simulink library "utilities"  (R2016b)
settings: Solver=VariableStepAuto  StartTime=0.0  StopTime=10.0  RelTol=1e-3
settings Model: Creator=bclzl  LastModifiedBy=bclzl

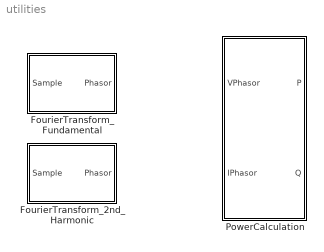
== system utilities ==
  FourierTransform_2nd_Harmonic : Subsystem
  FourierTransform_Fundamental : Subsystem
  PowerCalculation : Subsystem

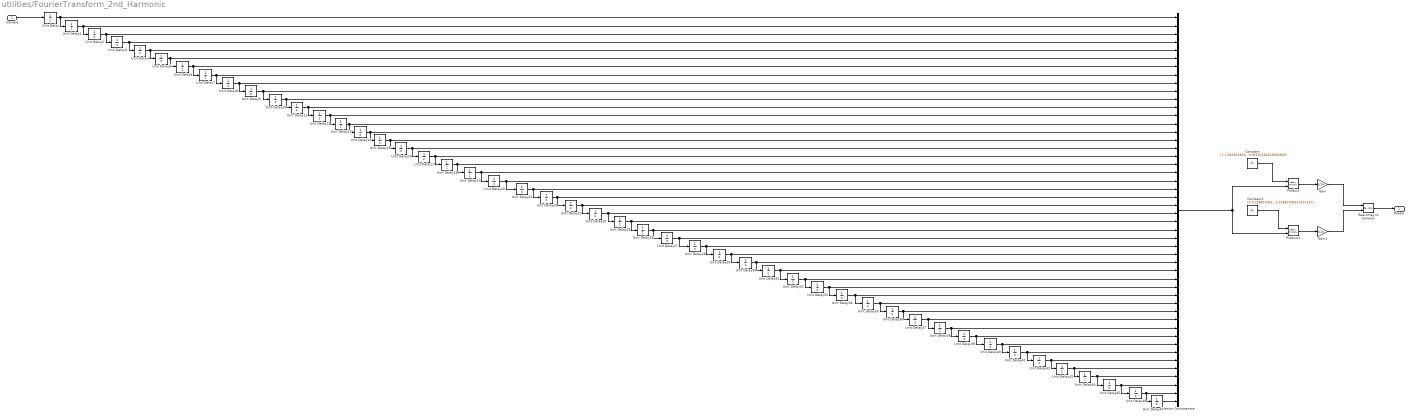
== system utilities/FourierTransform_2nd_Harmonic ==
  Sample : Inport
  Constant : Constant  Value=[1 0.96592582628906831 0.86602540378443871 0.70710678118654757 0.50000000000000011 0.25881904510252074 6.123233995736766E-17 -0.25881904510252063 -0.49999999999999978 -0.70710678118654746 -0.86602540378443871 -0.9659258262890682 -1 -0.96592582628906831 -0.86602540378443882 -0.70710678118654791 -0.50000000000000044 -0.25881904510252063 -1.8369701987210297E-16 0.2588190451025203 0.50000000000000011 0.70710678118654735 0.86602540378443837 0.96592582628906809 1 0.96592582628906831 0.86602540378443871 0.70710678118654757 0.50000000000000011 0.25881904510252074 6.123233995736766E-17 -0.25881904510252063 -0.49999999999999978 -0.70710678118654746 -0.86602540378443871 -0.9659258262890682 -1 -0.96592582628906831 -0.86602540378443882 -0.70710678118654791 -0.50000000000000044 -0.25881904510252063 -1.8369701987210297E-16 0.2588190451025203 0.50000000000000011 0.70710678118654735 0.86602540378443837 0.96592582628906809]  VectorParams1D=off
  Constant1 : Constant  Value=[0 0.25881904510252074 0.49999999999999994 0.70710678118654746 0.8660254037844386 0.96592582628906831 1 0.96592582628906831 0.86602540378443871 0.70710678118654757 0.49999999999999994 0.258819045102521 1.2246467991473532E-16 -0.25881904510252079 -0.49999999999999972 -0.70710678118654713 -0.86602540378443849 -0.96592582628906831 -1 -0.96592582628906842 -0.8660254037844386 -0.70710678118654768 -0.50000000000000044 -0.25881904510252157 0 0.25881904510252074 0.49999999999999994 0.70710678118654746 0.8660254037844386 0.96592582628906831 1 0.96592582628906831 0.86602540378443871 0.70710678118654757 0.49999999999999994 0.258819045102521 1.2246467991473532E-16 -0.25881904510252079 -0.49999999999999972 -0.70710678118654713 -0.86602540378443849 -0.96592582628906831 -1 -0.96592582628906842 -0.8660254037844386 -0.70710678118654768 -0.50000000000000044 -0.25881904510252157]  VectorParams1D=off
  Gain : Gain  Gain=1/24
  Gain1 : Gain  Gain=1/24
  Product : Product  Multiplication=Matrix(*)
  Product1 : Product  Multiplication=Matrix(*)
  Real-Imag to Complex : RealImagToComplex
  Unit Delay{,1..47} (48 alike) : UnitDelay  SampleTime=-1
  Vector Concatenate : Concatenate  NumInputs=48  Mode=Multidimensional array
  Phasor : Outport
  wires:
  Real-Imag to Complex/1 -> Phasor/1
  Gain1/1 -> Real-Imag to Complex/2
  Product1/1 -> Gain1/1
  Constant1/1 -> Product1/1
  Gain/1 -> Real-Imag to Complex/1
  Product/1 -> Gain/1
  Constant/1 -> Product/1
  Unit Delay29/1 -> Unit Delay30/1, Vector Concatenate/30
  Unit Delay30/1 -> Unit Delay31/1, Vector Concatenate/31
  Unit Delay26/1 -> Unit Delay27/1, Vector Concatenate/27
  Unit Delay27/1 -> Unit Delay28/1, Vector Concatenate/28
  Unit Delay28/1 -> Unit Delay29/1, Vector Concatenate/29
  Unit Delay41/1 -> Unit Delay42/1, Vector Concatenate/42
  Unit Delay42/1 -> Unit Delay43/1, Vector Concatenate/43
  Unit Delay43/1 -> Unit Delay44/1, Vector Concatenate/44
  Unit Delay46/1 -> Unit Delay47/1, Vector Concatenate/47
  Unit Delay40/1 -> Unit Delay41/1, Vector Concatenate/41
  Unit Delay47/1 -> Vector Concatenate/48
  Sample/1 -> Unit Delay/1
  Unit Delay1/1 -> Unit Delay2/1, Vector Concatenate/2
  Vector Concatenate/1 -> Product/2, Product1/2
  Unit Delay5/1 -> Unit Delay6/1, Vector Concatenate/6
  Unit Delay19/1 -> Unit Delay20/1, Vector Concatenate/20
  Unit Delay20/1 -> Unit Delay21/1, Vector Concatenate/21
  Unit Delay21/1 -> Unit Delay22/1, Vector Concatenate/22
  Unit Delay24/1 -> Unit Delay25/1, Vector Concatenate/25
  Unit Delay23/1 -> Unit Delay24/1, Vector Concatenate/24
  Unit Delay22/1 -> Unit Delay23/1, Vector Concatenate/23
  Unit Delay9/1 -> Unit Delay10/1, Vector Concatenate/10
  Unit Delay25/1 -> Unit Delay26/1, Vector Concatenate/26
  Unit Delay13/1 -> Unit Delay14/1, Vector Concatenate/14
  Unit Delay6/1 -> Unit Delay7/1, Vector Concatenate/7
  Unit Delay4/1 -> Unit Delay5/1, Vector Concatenate/5
  Unit Delay14/1 -> Unit Delay15/1, Vector Concatenate/15
  Unit Delay17/1 -> Unit Delay18/1, Vector Concatenate/18
  Unit Delay16/1 -> Unit Delay17/1, Vector Concatenate/17
  Unit Delay18/1 -> Unit Delay19/1, Vector Concatenate/19
  Unit Delay15/1 -> Unit Delay16/1, Vector Concatenate/16
  Unit Delay8/1 -> Unit Delay9/1, Vector Concatenate/9
  Unit Delay3/1 -> Unit Delay4/1, Vector Concatenate/4
  Unit Delay2/1 -> Unit Delay3/1, Vector Concatenate/3
  Unit Delay12/1 -> Unit Delay13/1, Vector Concatenate/13
  Unit Delay10/1 -> Unit Delay11/1, Vector Concatenate/11
  Unit Delay11/1 -> Unit Delay12/1, Vector Concatenate/12
  Unit Delay/1 -> Unit Delay1/1, Vector Concatenate/1
  Unit Delay37/1 -> Unit Delay38/1, Vector Concatenate/38
  Unit Delay38/1 -> Unit Delay39/1, Vector Concatenate/39
  Unit Delay39/1 -> Unit Delay40/1, Vector Concatenate/40
  Unit Delay34/1 -> Unit Delay35/1, Vector Concatenate/35
  Unit Delay35/1 -> Unit Delay36/1, Vector Concatenate/36
  Unit Delay36/1 -> Unit Delay37/1, Vector Concatenate/37
  Unit Delay33/1 -> Unit Delay34/1, Vector Concatenate/34
  Unit Delay32/1 -> Unit Delay33/1, Vector Concatenate/33
  Unit Delay44/1 -> Unit Delay45/1, Vector Concatenate/45
  Unit Delay45/1 -> Unit Delay46/1, Vector Concatenate/46
  Unit Delay7/1 -> Unit Delay8/1, Vector Concatenate/8
  Unit Delay31/1 -> Unit Delay32/1, Vector Concatenate/32

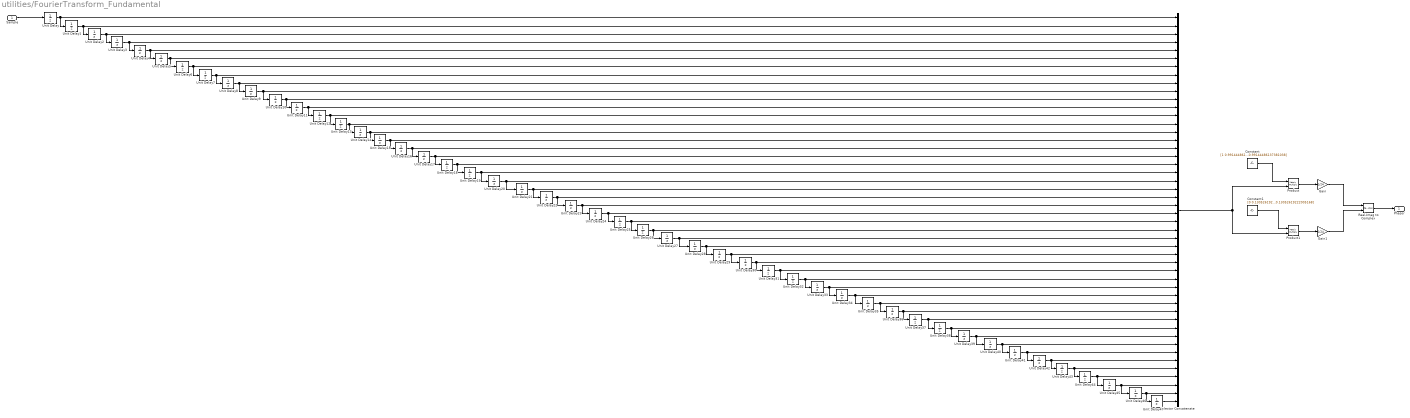
== system utilities/FourierTransform_Fundamental ==
  Sample : Inport
  Constant : Constant  Value=[1 0.99144486137381038 0.96592582628906831 0.92387953251128674 0.86602540378443871 0.79335334029123517 0.70710678118654757 0.60876142900872066 0.50000000000000011 0.38268343236508984 0.25881904510252074 0.13052619222005171 6.123233995736766E-17 -0.13052619222005138 -0.25881904510252085 -0.38268343236508973 -0.49999999999999978 -0.60876142900872066 -0.70710678118654746 -0.793353340291235 -0.86602540378443871 -0.92387953251128674 -0.9659258262890682 -0.99144486137381038 -1 -0.99144486137381038 -0.96592582628906842 -0.92387953251128685 -0.8660254037844386 -0.79335334029123539 -0.70710678118654768 -0.60876142900872088 -0.50000000000000044 -0.38268343236509034 -0.25881904510252063 -0.13052619222005163 -1.8369701987210297E-16 0.13052619222005127 0.2588190451025203 0.38268343236509 0.50000000000000011 0.60876142900872054 0.70710678118654735 0.79335334029123494 0.86602540378443837 0.92387953251128652 0.96592582628906831 0.99144486137381038]  VectorParams1D=off
  Constant1 : Constant  Value=[0 0.13052619222005157 0.25881904510252074 0.38268343236508978 0.49999999999999994 0.60876142900872066 0.70710678118654746 0.79335334029123517 0.8660254037844386 0.92387953251128674 0.96592582628906831 0.99144486137381038 1 0.99144486137381049 0.96592582628906831 0.92387953251128674 0.86602540378443871 0.79335334029123517 0.70710678118654757 0.60876142900872088 0.49999999999999994 0.38268343236508989 0.258819045102521 0.13052619222005157 1.2246467991473532E-16 -0.13052619222005177 -0.25881904510252035 -0.38268343236508967 -0.50000000000000011 -0.60876142900872032 -0.70710678118654746 -0.79335334029123494 -0.86602540378443849 -0.92387953251128652 -0.96592582628906831 -0.99144486137381038 -1 -0.99144486137381049 -0.96592582628906842 -0.92387953251128663 -0.8660254037844386 -0.79335334029123517 -0.70710678118654768 -0.60876142900872088 -0.50000000000000044 -0.38268343236509039 -0.25881904510252068 -0.13052619222005168]  VectorParams1D=off
  Gain : Gain  Gain=1/24
  Gain1 : Gain  Gain=1/24
  Product : Product  Multiplication=Matrix(*)
  Product1 : Product  Multiplication=Matrix(*)
  Real-Imag to Complex : RealImagToComplex
  Unit Delay{,1..47} (48 alike) : UnitDelay  SampleTime=-1
  Vector Concatenate : Concatenate  NumInputs=48  Mode=Multidimensional array
  Phasor : Outport
  wires:
  Unit Delay31/1 -> Vector Concatenate/32, Unit Delay32/1
  Unit Delay7/1 -> Vector Concatenate/8, Unit Delay8/1
  Unit Delay45/1 -> Vector Concatenate/46, Unit Delay46/1
  Unit Delay44/1 -> Vector Concatenate/45, Unit Delay45/1
  Unit Delay32/1 -> Vector Concatenate/33, Unit Delay33/1
  Unit Delay33/1 -> Vector Concatenate/34, Unit Delay34/1
  Unit Delay36/1 -> Vector Concatenate/37, Unit Delay37/1
  Unit Delay35/1 -> Vector Concatenate/36, Unit Delay36/1
  Unit Delay34/1 -> Vector Concatenate/35, Unit Delay35/1
  Unit Delay39/1 -> Vector Concatenate/40, Unit Delay40/1
  Unit Delay38/1 -> Vector Concatenate/39, Unit Delay39/1
  Unit Delay37/1 -> Vector Concatenate/38, Unit Delay38/1
  Unit Delay/1 -> Vector Concatenate/1, Unit Delay1/1
  Unit Delay11/1 -> Vector Concatenate/12, Unit Delay12/1
  Unit Delay10/1 -> Vector Concatenate/11, Unit Delay11/1
  Unit Delay12/1 -> Vector Concatenate/13, Unit Delay13/1
  Unit Delay2/1 -> Vector Concatenate/3, Unit Delay3/1
  Unit Delay3/1 -> Vector Concatenate/4, Unit Delay4/1
  Unit Delay8/1 -> Vector Concatenate/9, Unit Delay9/1
  Unit Delay15/1 -> Vector Concatenate/16, Unit Delay16/1
  Unit Delay18/1 -> Vector Concatenate/19, Unit Delay19/1
  Unit Delay16/1 -> Vector Concatenate/17, Unit Delay17/1
  Unit Delay17/1 -> Vector Concatenate/18, Unit Delay18/1
  Unit Delay14/1 -> Vector Concatenate/15, Unit Delay15/1
  Unit Delay4/1 -> Vector Concatenate/5, Unit Delay5/1
  Unit Delay6/1 -> Vector Concatenate/7, Unit Delay7/1
  Unit Delay13/1 -> Vector Concatenate/14, Unit Delay14/1
  Unit Delay25/1 -> Vector Concatenate/26, Unit Delay26/1
  Unit Delay9/1 -> Vector Concatenate/10, Unit Delay10/1
  Unit Delay22/1 -> Vector Concatenate/23, Unit Delay23/1
  Unit Delay23/1 -> Vector Concatenate/24, Unit Delay24/1
  Unit Delay24/1 -> Vector Concatenate/25, Unit Delay25/1
  Unit Delay21/1 -> Vector Concatenate/22, Unit Delay22/1
  Unit Delay20/1 -> Vector Concatenate/21, Unit Delay21/1
  Unit Delay19/1 -> Vector Concatenate/20, Unit Delay20/1
  Unit Delay5/1 -> Vector Concatenate/6, Unit Delay6/1
  Vector Concatenate/1 -> Product1/2, Product/2
  Unit Delay1/1 -> Vector Concatenate/2, Unit Delay2/1
  Sample/1 -> Unit Delay/1
  Unit Delay47/1 -> Vector Concatenate/48
  Unit Delay40/1 -> Vector Concatenate/41, Unit Delay41/1
  Unit Delay46/1 -> Vector Concatenate/47, Unit Delay47/1
  Unit Delay43/1 -> Vector Concatenate/44, Unit Delay44/1
  Unit Delay42/1 -> Vector Concatenate/43, Unit Delay43/1
  Unit Delay41/1 -> Vector Concatenate/42, Unit Delay42/1
  Unit Delay28/1 -> Vector Concatenate/29, Unit Delay29/1
  Unit Delay27/1 -> Vector Concatenate/28, Unit Delay28/1
  Unit Delay26/1 -> Vector Concatenate/27, Unit Delay27/1
  Unit Delay30/1 -> Vector Concatenate/31, Unit Delay31/1
  Unit Delay29/1 -> Vector Concatenate/30, Unit Delay30/1
  Constant/1 -> Product/1
  Product/1 -> Gain/1
  Gain/1 -> Real-Imag to Complex/1
  Constant1/1 -> Product1/1
  Product1/1 -> Gain1/1
  Gain1/1 -> Real-Imag to Complex/2
  Real-Imag to Complex/1 -> Phasor/1

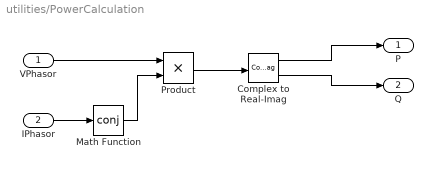
== system utilities/PowerCalculation ==
  VPhasor : Inport
  IPhasor : Inport  Port=2
  Complex to Real-Imag : ComplexToRealImag
  Math Function : Math  Operator=conj  SaturateOnIntegerOverflow=on
  Product : Product
  P : Outport
  Q : Outport  Port=2
  wires:
  VPhasor/1 -> Product/1
  IPhasor/1 -> Math Function/1
  Math Function/1 -> Product/2
  Product/1 -> Complex to Real-Imag/1
  Complex to Real-Imag/1 -> P/1
  Complex to Real-Imag/2 -> Q/1
